simulink library "Project1_Library"  (R2017b)
settings: Solver=VariableStepAuto  StartTime=0.0  StopTime=10.0  RelTol=1e-3
settings Model: Creator=hattanbadyah  LastModifiedBy=hattanbadyah

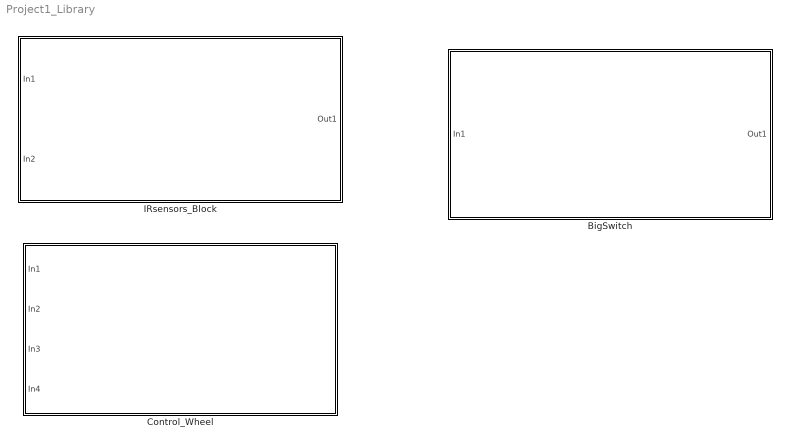
== system Project1_Library ==
  BigSwitch : Subsystem
      mask Help: Click on this link for more information:
      mask Display:
      | disp('BigSwitch');
      | port_label('output',1,'BigSwitch');
      | port_label('input', 1,'manual_switch');
  Control_Wheel : Subsystem
      mask Help: Click on this link for more information:
      mask Display:
      | disp('Control_Wheel');
      | port_label('input', 1,'LeftW');
      | port_label('input', 2,'RightW');
      | port_label('input', 3,'TurnWheel');
      | port_label('input', 4,'BigSwitch');
  IRsensors_Block : Subsystem
      mask Help: Click on this link for more information
      mask Display:
      | disp('IRsensors_Block');
      | port_label('input',1,'ReadSensor');
      | port_label('input', 2,'BigSwitch');
      | port_label('output', 1,'SensorsRead');

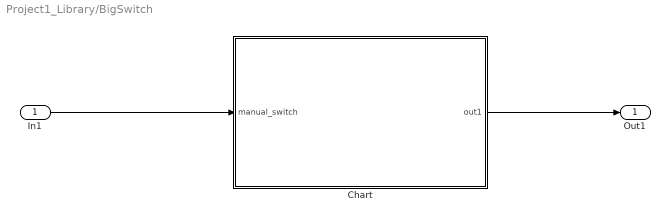
== system Project1_Library/BigSwitch ==
  In1 : Inport
  Chart : Stateflow chart  TreatAsAtomicUnit=on
  Out1 : Outport
  wires:
  In1/1 -> Chart/1(manual_switch)
  Chart/1(out1) -> Out1/1

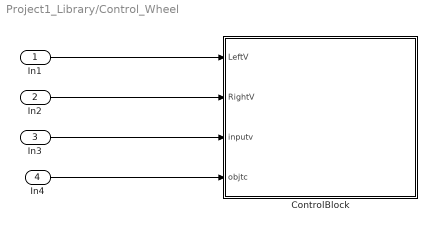
== system Project1_Library/Control_Wheel ==
  In1 : Inport
  In2 : Inport  Port=2
  In3 : Inport  Port=3
  In4 : Inport  Port=4
  ControlBlock : Stateflow chart  TreatAsAtomicUnit=on
  wires:
  In1/1 -> ControlBlock/1(LeftV)
  In2/1 -> ControlBlock/2(RightV)
  In3/1 -> ControlBlock/3(inputv)
  In4/1 -> ControlBlock/4(objtc)

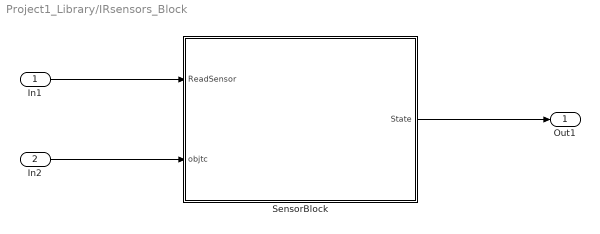
== system Project1_Library/IRsensors_Block ==
  In1 : Inport
  In2 : Inport  Port=2
  SensorBlock : Stateflow chart  TreatAsAtomicUnit=on
  Out1 : Outport
  wires:
  In1/1 -> SensorBlock/1(ReadSensor)
  In2/1 -> SensorBlock/2(objtc)
  SensorBlock/1(State) -> Out1/1

== stateflow chart Project1_Library/IRsensors_Block/SensorBlock ==
  state A
  state Start
    entry, during:
    coder.extrinsic('evalin')
    so=evalin('base','objWs');
    %status = 0
  state Sensor
    entry, during:
    coder.extrinsic('RangeStateRoomba');
    State=RangeStateRoomba(so);
    %status = 1;
  (default) -> A
  A -> Start : [objtc==1]
  Start -> Sensor : [ReadSensor==1]
  Sensor -> Start : [ReadSensor==0]
  data: ReadSensor input; so local; State output double size=6; objtc input

== stateflow chart Project1_Library/BigSwitch/Chart ==
  state A
    en,du:
    tcpInit;
    out1 = 1;
  state Connect
    entry:
    y=1
  state Disconnect
    entry: coder.extrinsic('evalin');
    so=evalin('base','objWs');
    fclose(so);
  state Refresh
    entry:
    y = y + 1
    if y==3
    y = 1
    end
  (default) -> A
  Disconnect -> A : [manual_switch==1]
  A -> Connect : [manual_switch==1]
  Connect -> Refresh : [manual_switch==1]
  Refresh -> Connect [order 1] : [manual_switch==1]
  Refresh -> Disconnect [order 2] : [manual_switch==0]
  data: out1 output; manual_switch input; y local; so local
  function tcpInit:
    | function tcpInit
    | coder.extrinsic('tcpip');
    | coder.extrinsic('assignin');
    | persistent obj
    | if isempty(obj)
    |     obj=tcpip('10.0.0.1',9001);
    |     set(obj,'Terminator','LF')
    |     set(obj,'InputBufferSize',1000)
    |     set(obj, 'Timeout', .5)
    |     set(obj, 'ByteOrder','bigEndian');
    |     assignin('base','objWs',obj);
    |     
    | fopen(obj);
    |     % Start!
    | Start=[128];
    | fwrite(obj,Start);
    | pause(.1)
    | Mode=[132]
    | fwrite(obj,Mode);
    | pause(.1)
    | 
    | % %Print 'go' on display
    | fwrite(obj, [164, 71, 79, 32, 32]);
    | % make a sound
    | fwrite(obj, [140 1 3 60 20 72 20 84 40 ]); %RoombaInit Song
    | fwrite(obj, [140 2 1 60 20]); % BeepRoomba song
    | fwrite(obj, [140 3 3 84 20 72 30 60 40]); % PowerOffRoomba song
    | fwrite(obj, [141 1]); % play RoombaInit song
    | disp('Robot should display go on 7 segment LED panel and play song.')
    | pause(1);
    | end

== stateflow chart Project1_Library/Control_Wheel/ControlBlock ==
  state blank
  state Connect
    entry:
    coder.extrinsic('evalin');
    obj=evalin('base','objWs');
    %status= 0
  state Reset_Stop
    entry:
    coder.extrinsic('SetWheelVelRoomba')
    SetWheelVelRoomba(obj,0, 0)
    %status=2
  state Update
    entry,during:
    coder.extrinsic('SetWheelVelRoomba')
    SetWheelVelRoomba(obj,RightV, LeftV)
    %status=1
  state start
    entry,during:
    coder.extrinsic('SetWheelVelRoomba')
    SetWheelVelRoomba(obj,RightV, LeftV)
    %status=1
  (default) -> blank
  blank -> Connect : [objtc==1]
  Reset_Stop -> Connect [order 2] : after(30,sec)
  Connect -> start : [inputv==1]
  Update -> start : after(0.5,sec)
  start -> Reset_Stop [order 1] : [inputv==0]
  Reset_Stop -> start [order 1] : [inputv==1]
  start -> Update [order 2] : after(0.5,sec)
  data: LeftV input; RightV input; inputv input; objtc input; obj local
